simulink model "massSpringDamper"  (R2022a)
settings: Solver=VariableStepAuto  StartTime=0.0  StopTime=10.0  RelTol=1e-3
undefined symbols (not defined in the file or in its folder): c1, c2, d2, m1, m2
settings Model: Creator=Anwender  LastModifiedBy=Anwender

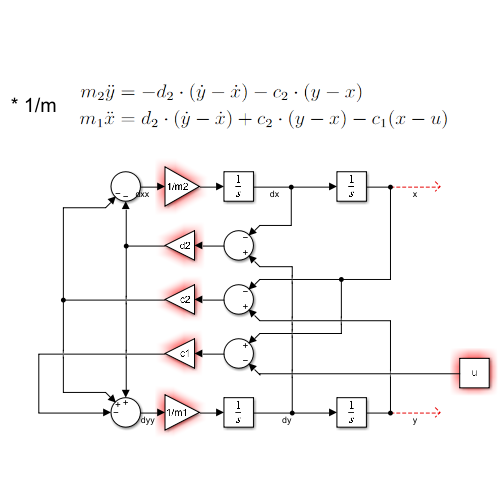
[thumbnail: Simulink's stored preview of the top-level diagram]
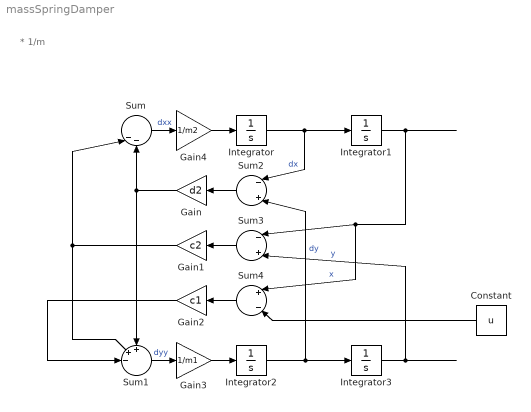
== system massSpringDamper ==
  note: * 1/m
  Constant : Constant  Value=u
  Gain : Gain  Gain=d2
  Gain1 : Gain  Gain=c2
  Gain2 : Gain  Gain=c1
  Gain3 : Gain  Gain=1/m1
  Gain4 : Gain  Gain=1/m2
  Integrator{,1..3} (4 alike) : Integrator
  Sum : Sum  Inputs=|||--
  Sum1 : Sum  Inputs=++-||
  Sum2 : Sum  Inputs=|-|+|
  Sum3 : Sum  Inputs=|-|+|
  Sum4 : Sum  Inputs=|+|-|
  wires:
  Integrator/1 -> Sum2/1, Integrator1/1  "dx"
  Sum/1 -> Gain4/1  "dxx"
  Integrator1/1 -> Sum4/1, Sum3/1  "x"
  Integrator3/1 -> Sum3/2  "y"
  Sum1/1 -> Gain3/1  "dyy"
  Integrator2/1 -> Integrator3/1, Sum2/2  "dy"
  Gain2/1 -> Sum1/3
  Gain1/1 -> Sum/1, Sum1/2
  Gain/1 -> Sum1/1, Sum/2
  Sum2/1 -> Gain/1
  Sum3/1 -> Gain1/1
  Sum4/1 -> Gain2/1
  Constant/1 -> Sum4/2
  Gain3/1 -> Integrator2/1
  Gain4/1 -> Integrator/1
